simulink model "FM_SIM"  (R2024a)
settings: Solver=VariableStepAuto  StartTime=0.0  StopTime=10.0  RelTol=1e-3
libraries: dspfdesign x4
settings Model: Creator=adity  LastModifiedBy=adity

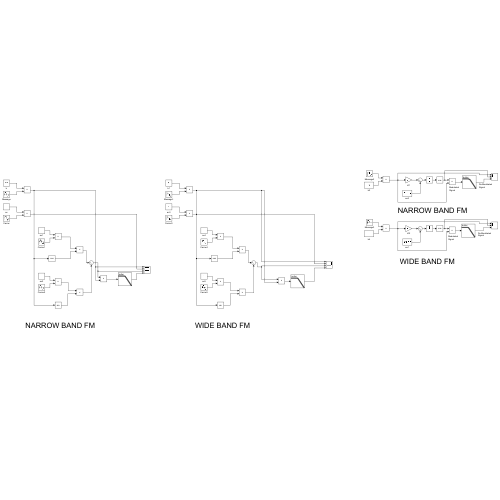
[thumbnail: Simulink's stored preview of the top-level diagram]
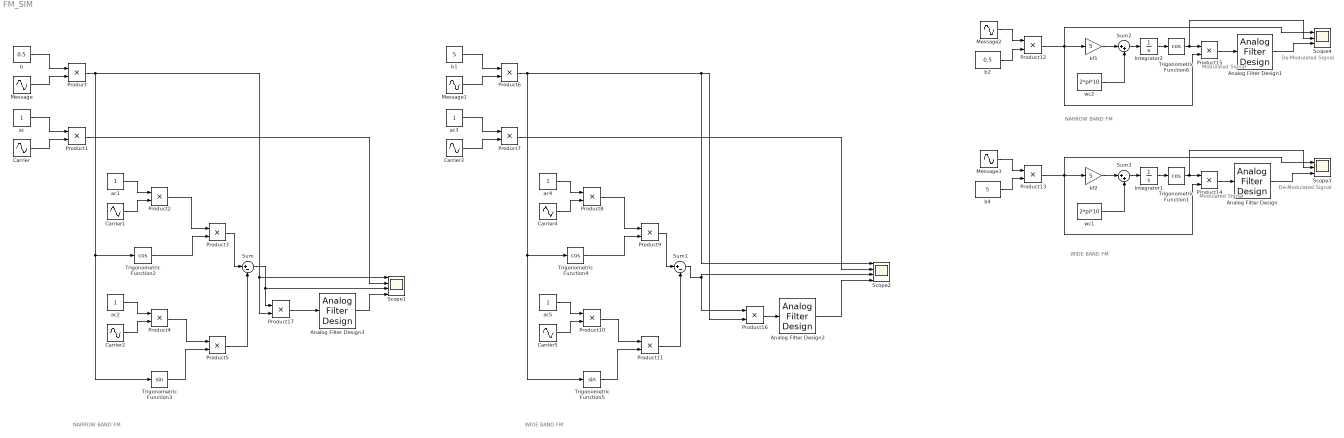
== system FM_SIM ==
  note: Modulated
      | Signal
  note: NARROW BAND FM
  note: WIDE BAND FM
  note: WIDE BAND FM
  note: NARROW BAND FM
  note: De-Modulated
      | Signal
  note: De-Modulated
      | Signal
  note: Modulated
      | Signal
  Analog Filter Design : dspfdesign/Analog Filter Design  method=Butterworth  filttype=Lowpass  N=10  Wlo=2*pi*1  Whi=80  Rp=2  Rs=40
  Analog Filter Design1 : dspfdesign/Analog Filter Design  method=Butterworth  filttype=Lowpass  N=3  Wlo=2*pi*1  Whi=80  Rp=2  Rs=40
  Analog Filter Design2 : dspfdesign/Analog Filter Design  method=Butterworth  filttype=Lowpass  N=10  Wlo=2*pi*1  Whi=80  Rp=2  Rs=40
  Analog Filter Design3 : dspfdesign/Analog Filter Design  method=Butterworth  filttype=Lowpass  N=10  Wlo=2*pi*1  Whi=80  Rp=2  Rs=40
  Carrier{,1,3..4} (4 alike) : Sin  Frequency=2*pi*10  Phase=pi/2  SampleTime=1/1000
  Carrier2 : Sin  Frequency=2*pi*10  SampleTime=1/1000
  Carrier5 : Sin  Frequency=2*pi*10  SampleTime=1/1000
  Integrator1 : Integrator
  Integrator2 : Integrator
  Message{,1..3} (4 alike) : Sin  Frequency=2*pi*1  SampleTime=1/1000
  Product{,1..17} (18 alike) : Product
  Scope1 : Scope  NumInputPorts=4
  Scope2 : Scope  NumInputPorts=4
  Scope3 : Scope  NumInputPorts=3
  Scope4 : Scope  NumInputPorts=3
  Sum : Sum  Inputs=|+-
  Sum1 : Sum  Inputs=|+-
  Sum2 : Sum  Inputs=|++
  Sum3 : Sum  Inputs=|++
  Trigonometric Function{1..2,4,6} (4 alike) : Trigonometry  Operator=cos
  Trigonometric Function3 : Trigonometry
  Trigonometric Function5 : Trigonometry
  ac{,1..5} (6 alike) : Constant
  b : Constant  Value=0.5
  b1 : Constant  Value=5
  b2 : Constant  Value=0.5
  b4 : Constant  Value=5
  kf1 : Gain  Gain=5
  kf2 : Gain  Gain=5
  wc1 : Constant  Value=2*pi*10
  wc2 : Constant  Value=2*pi*10
  wires:
  kf2/1 -> Sum3/1
  Carrier3/1 -> Product7/2
  Product13/1 -> Product14/2, kf2/1, Scope3/1
  Product/1 -> Product17/2, Scope1/1, Trigonometric Function3/1, Trigonometric Function2/1
  ac/1 -> Product1/1
  b/1 -> Product/1
  Product5/1 -> Sum/2
  b4/1 -> Product13/2
  Carrier1/1 -> Product2/2
  ac2/1 -> Product4/1
  Product2/1 -> Product3/1
  Trigonometric Function2/1 -> Product3/2
  ac1/1 -> Product2/1
  Sum1/1 -> Product16/1, Scope2/3
  Product1/1 -> Scope1/2
  Sum/1 -> Product17/1, Scope1/3
  Message/1 -> Product/2
  Product4/1 -> Product5/1
  Product6/1 -> Product16/2, Scope2/1, Trigonometric Function5/1, Trigonometric Function4/1
  Trigonometric Function5/1 -> Product11/2
  Carrier5/1 -> Product10/2
  Product3/1 -> Sum/1
  ac3/1 -> Product7/1
  b1/1 -> Product6/1
  Message3/1 -> Product13/1
  Product11/1 -> Sum1/2
  Product7/1 -> Scope2/2
  Trigonometric Function3/1 -> Product5/2
  Product9/1 -> Sum1/1
  Carrier/1 -> Product1/2
  Carrier2/1 -> Product4/2
  Product10/1 -> Product11/1
  Integrator1/1 -> Trigonometric Function1/1
  Sum3/1 -> Integrator1/1
  wc1/1 -> Sum3/2
  ac4/1 -> Product8/1
  ac5/1 -> Product10/1
  Product8/1 -> Product9/1
  Message1/1 -> Product6/2
  Carrier4/1 -> Product8/2
  Trigonometric Function4/1 -> Product9/2
  Product14/1 -> Analog Filter Design/1
  Trigonometric Function1/1 -> Scope3/2, Product14/1
  Analog Filter Design/1 -> Scope3/3
  Trigonometric Function6/1 -> Scope4/2, Product15/1
  Analog Filter Design1/1 -> Scope4/3
  Product15/1 -> Analog Filter Design1/1
  b2/1 -> Product12/2
  wc2/1 -> Sum2/2
  Message2/1 -> Product12/1
  Product12/1 -> Product15/2, kf1/1, Scope4/1
  Integrator2/1 -> Trigonometric Function6/1
  kf1/1 -> Sum2/1
  Sum2/1 -> Integrator2/1
  Product16/1 -> Analog Filter Design2/1
  Analog Filter Design2/1 -> Scope2/4
  Analog Filter Design3/1 -> Scope1/4
  Product17/1 -> Analog Filter Design3/1
